simulink library "thermostat"  (R2024b)
settings: Solver=VariableStepAuto  StartTime=0.0  StopTime=10.0  RelTol=1e-3
settings Model: Creator=fergusproctor  LastModifiedBy=fergusproctor

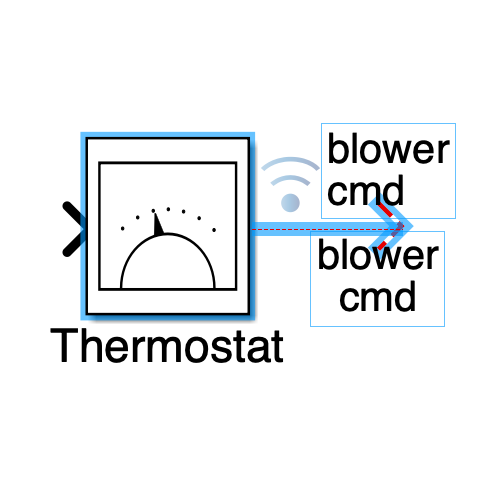
[thumbnail: Simulink's stored preview of the top-level diagram]
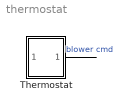
== system thermostat ==
  Thermostat : Subsystem
      mask Display: image('HouseHeatThermostatPix.svg')
  wires:
  Thermostat/1(Blower switch) -> ?  "blower cmd"

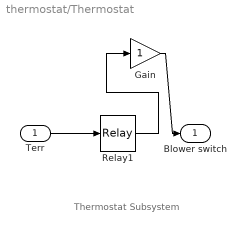
== system thermostat/Thermostat ==
  note: Thermostat Subsystem
  Terr : Inport
  Gain : Gain
  Relay1 : Relay  OnSwitchValue=2  OffSwitchValue=-2
  Blower switch : Outport  InitialOutput=0  VectorParamsAs1DForOutWhenUnconnected=off
  wires:
  Terr/1 -> Relay1/1
  Relay1/1 -> Gain/1
  Gain/1 -> Blower switch/1
